simulink model "chap1_7"  (R2023b)
settings: Solver=ode4  StartTime=0.0  StopTime=1  RelTol=1e-3  EnableMultiTasking=on
undefined symbols (not defined in the file or in its folder): chap1_7ctrl
settings Model: Creator=CorgiQvm  LastModifiedBy=CorgiQvm
settings DataIOCC: Decimation=100  SaveFormat=Array  SaveOutput=off  SaveTime=off  ReturnWorkspaceOutputs=off

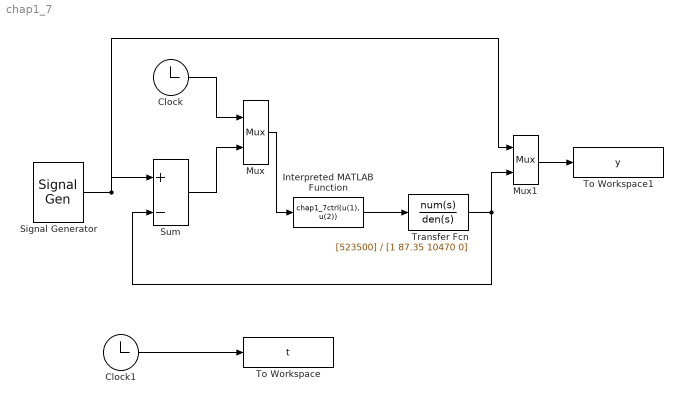
== system chap1_7 ==
  Clock : Clock
  Clock1 : Clock
  Interpreted MATLAB Function : MATLABFcn  MATLABFcn=chap1_7ctrl(u(1), u(2))
  Mux : Mux  Inputs=2
  Mux1 : Mux  Inputs=2
  Signal Generator : SignalGenerator  Amplitude=0.05
  Sum : Sum  Inputs=|+-  InputSameDT=on  SaturateOnIntegerOverflow=on  OutDataTypeStr=Inherit: Same as first input
  To Workspace : ToWorkspace  VariableName=t  SampleTime=-1
  To Workspace1 : ToWorkspace  VariableName=y  SampleTime=-1
  Transfer Fcn : TransferFcn  Numerator=[523500]  Denominator=[1 87.35 10470 0]
  wires:
  Mux1/1 -> To Workspace1/1
  Clock1/1 -> To Workspace/1
  Signal Generator/1 -> Mux1/1, Sum/1
  Sum/1 -> Mux/2
  Clock/1 -> Mux/1
  Mux/1 -> Interpreted MATLAB Function/1
  Interpreted MATLAB Function/1 -> Transfer Fcn/1
  Transfer Fcn/1 -> Sum/2, Mux1/2
